simulink library "PropLoads"  (R2024a)
settings: Solver=VariableStepAuto  StartTime=0.0  StopTime=10.0  RelTol=1e-3
undefined symbols (not defined in the file): m1_fail, m2_fail, m3_fail, m4_fail, r1, r2, r3, r4
libraries: matrix_library x4, MT3515 x4, simulink_extras x2, aerolibatmos2 x1, aerolibasang x1
settings Model: Creator=igmso  LastModifiedBy=igmso

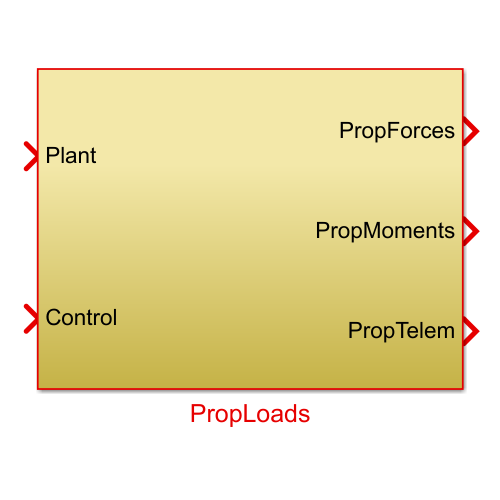
[thumbnail: Simulink's stored preview of the top-level diagram]
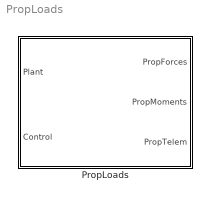
== system PropLoads ==
  PropLoads : Subsystem

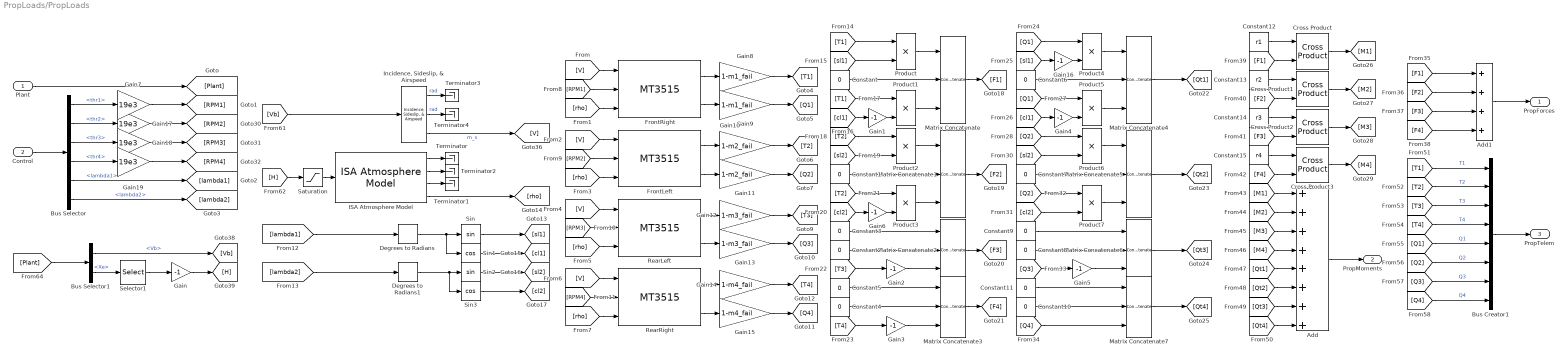
== system PropLoads/PropLoads ==
  Plant : Inport
  Control : Inport  Port=2
  Add : Sum  Inputs=8
  Add1 : Sum  Inputs=4
  Bus Creator1 : BusCreator  Inputs=8
  Bus Selector : BusSelector  OutputSignals=thr1,thr2,thr3,thr4,lambda1,lambda2
  Bus Selector1 : BusSelector  OutputSignals=Vb,Xe
  Constant{,1..11} (12 alike) : Constant  Value=0  SampleTime=-1
  Constant12 : Constant  Value=r1  SampleTime=-1
  Constant13 : Constant  Value=r2  SampleTime=-1
  Constant14 : Constant  Value=r3  SampleTime=-1
  Constant15 : Constant  Value=r4  SampleTime=-1
  Cross Product{,1..3} (4 alike) : matrix_library/Cross Product
  Degrees to Radians : simulink_extras/Transformations/Degrees to Radians
  Degrees to Radians1 : simulink_extras/Transformations/Degrees to Radians
  FrontLeft : MT3515/MT3515  SystemSampleTime=-1  VariantActivationTime=update diagram  AllowFlexibleInterface=on  Latency=0  AutoFrameSizeCalculation=off
  FrontRight : MT3515/MT3515  SystemSampleTime=-1  VariantActivationTime=update diagram  AllowFlexibleInterface=on  Latency=0  AutoFrameSizeCalculation=off
  Gain{,1..6,16} (8 alike) : Gain  Gain=-1
  Gain10 : Gain  Gain=1-m2_fail
  Gain11 : Gain  Gain=1-m2_fail
  Gain12 : Gain  Gain=1-m3_fail
  Gain13 : Gain  Gain=1-m3_fail
  Gain14 : Gain  Gain=1-m4_fail
  Gain15 : Gain  Gain=1-m4_fail
  Gain{7,17..19} (4 alike) : Gain  Gain=19e3
  Gain8 : Gain  Gain=1-m1_fail
  Gain9 : Gain  Gain=1-m1_fail
  ISA Atmosphere Model : aerolibatmos2/ISA Atmosphere Model  useExtended=off  action=Warning  custom=off  viscosityOut=off  g=9.80665  gamma=1.4  R=287.0531  L=0.0065  h_trop=11000  h_strat=20000  rho0=1.225  P0=101325  T0=288.15  h0=0  S=110.4  Tref=273.15  muref=1.716e-5
  "Incidence, Sideslip, & Airspeed" : aerolibasang/Incidence, Sideslip, & Airspeed
  Matrix Concatenate{,1..7} (8 alike) : Concatenate  NumInputs=3  ConcatenateDimension=2
  Product{,1..7} (8 alike) : Product
  RearLeft : MT3515/MT3515  SystemSampleTime=-1  VariantActivationTime=update diagram  AllowFlexibleInterface=on  Latency=0  AutoFrameSizeCalculation=off
  RearRight : MT3515/MT3515  SystemSampleTime=-1  VariantActivationTime=update diagram  AllowFlexibleInterface=on  Latency=0  AutoFrameSizeCalculation=off
  Saturation : Saturate  UpperLimit=20e3  LowerLimit=0
  Selector1 : Selector  InputPortWidth=3  IndexOptions=Index vector (dialog)  Indices=3  OutputSizes=1
  Sin : Trigonometry
  Sin1 : Trigonometry  Operator=cos
  Sin2 : Trigonometry
  Sin3 : Trigonometry  Operator=cos
  Terminator{,1..4} (5 alike) : Terminator
  PropForces : Outport
  PropMoments : Outport  Port=2
  PropTelem : Outport  Port=3
  wires:
  Saturation/1 -> ISA Atmosphere Model/1
  Gain19/1 -> [RPM4]
  Gain18/1 -> [RPM3]
  Gain17/1 -> [RPM2]
  Gain7/1 -> [RPM1]
  Gain16/1 -> Product4/2
  Gain14/1 -> [T4]
  Gain15/1 -> [Q4]
  Gain13/1 -> [Q3]
  Gain12/1 -> [T3]
  Gain11/1 -> [Q2]
  Gain10/1 -> [T2]
  Gain9/1 -> [Q1]
  Gain8/1 -> [T1]
  Product5/1 -> Matrix Concatenate4/3
  [RPM3] -> RearLeft/2
  Cross Product3/1 -> [M4]
  [rho] -> RearLeft/3
  FrontLeft/1 -> Gain10/1
  Constant12/1 -> Cross Product/1
  [T2] -> Product2/1
  [T3] -> Gain2/1
  [lambda2] -> Degrees to Radians1/1
  Sin1/1 -> [cl1]
  Matrix Concatenate1/1 -> [F2]
  [rho] -> FrontLeft/3
  [RPM4] -> RearRight/2
  FrontLeft/2 -> Gain11/1
  [RPM1] -> FrontRight/2
  Matrix Concatenate5/1 -> [Qt2]
  Bus Selector/1 -> Gain7/1  "<thr1>"
  Gain5/1 -> Matrix Concatenate6/3
  Sin3/1 -> [cl2]
  Matrix Concatenate7/1 -> [Qt4]
  [F1] -> Cross Product/2
  [V] -> FrontRight/1
  Gain4/1 -> Product5/2
  [cl2] -> Gain6/1
  [T1] -> Bus Creator1/1  "T1"
  [cl2] -> Product7/2
  [Q1] -> Product4/1
  [Qt3] -> Add/7
  Degrees to Radians1/1 -> Sin3/1, Sin2/1
  [lambda1] -> Degrees to Radians/1
  [sl2] -> Product6/2
  [M4] -> Add/4
  [M2] -> Add/2
  [M1] -> Add/1
  RearRight/1 -> Gain14/1
  [rho] -> RearRight/3
  Product3/1 -> Matrix Concatenate1/3
  [M3] -> Add/3
  [RPM2] -> FrontLeft/2
  [Qt4] -> Add/8
  [T4] -> Gain3/1
  [Qt2] -> Add/6
  [Qt1] -> Add/5
  Matrix Concatenate/1 -> [F1]
  RearLeft/2 -> Gain13/1
  Bus Creator1/1 -> PropTelem/1
  [Q1] -> Product5/1
  Product4/1 -> Matrix Concatenate4/1
  [V] -> RearLeft/1
  [F1] -> Add1/1
  FrontRight/2 -> Gain9/1
  Constant15/1 -> Cross Product3/1
  [V] -> FrontLeft/1
  RearRight/2 -> Gain15/1
  RearLeft/1 -> Gain12/1
  [Q2] -> Product7/1
  Constant4/1 -> Matrix Concatenate3/2
  [V] -> RearRight/1
  Bus Selector/6 -> [lambda2]  "<lambda2>"
  [cl1] -> Gain4/1
  [F2] -> Cross Product1/2
  [T4] -> Bus Creator1/4  "T4"
  [rho] -> FrontRight/3
  Bus Selector/5 -> [lambda1]  "<lambda1>"
  Constant1/1 -> Matrix Concatenate1/2
  Product2/1 -> Matrix Concatenate1/1
  [Q3] -> Gain5/1
  [sl2] -> Product2/2
  Plant/1 -> [Plant]
  Cross Product2/1 -> [M3]
  [cl1] -> Gain1/1
  [T2] -> Product3/1
  Constant11/1 -> Matrix Concatenate7/1
  Degrees to Radians/1 -> Sin1/1, Sin/1
  Constant10/1 -> Matrix Concatenate7/2
  [Q4] -> Bus Creator1/8  "Q4"
  Matrix Concatenate6/1 -> [Qt3]
  Matrix Concatenate3/1 -> [F4]
  [Q4] -> Matrix Concatenate7/3
  Constant9/1 -> Matrix Concatenate6/1
  Constant8/1 -> Matrix Concatenate6/2
  Product6/1 -> Matrix Concatenate5/1
  [Q2] -> Product6/1
  Constant7/1 -> Matrix Concatenate5/2
  Matrix Concatenate4/1 -> [Qt1]
  Product7/1 -> Matrix Concatenate5/3
  [sl1] -> Gain16/1
  Constant6/1 -> Matrix Concatenate4/2
  [T1] -> Product1/1
  Add/1 -> PropMoments/1
  Product/1 -> Matrix Concatenate/1
  [F3] -> Cross Product2/2
  Constant/1 -> Matrix Concatenate/2
  Product1/1 -> Matrix Concatenate/3
  Gain3/1 -> Matrix Concatenate3/3
  Constant14/1 -> Cross Product2/1
  Constant5/1 -> Matrix Concatenate3/1
  [T2] -> Bus Creator1/2  "T2"
  [T3] -> Bus Creator1/3  "T3"
  [Q2] -> Bus Creator1/6  "Q2"
  [Q1] -> Bus Creator1/5  "Q1"
  [Q3] -> Bus Creator1/7  "Q3"
  Cross Product/1 -> [M1]
  [T1] -> Product/1
  [F4] -> Cross Product3/2
  FrontRight/1 -> Gain8/1
  [sl1] -> Product/2
  Gain1/1 -> Product1/2
  [F2] -> Add1/2
  [F3] -> Add1/3
  [F4] -> Add1/4
  Cross Product1/1 -> [M2]
  Sin/1 -> [sl1]
  Constant3/1 -> Matrix Concatenate2/1
  Constant2/1 -> Matrix Concatenate2/2
  Matrix Concatenate2/1 -> [F3]
  Sin2/1 -> [sl2]
  Constant13/1 -> Cross Product1/1
  Add1/1 -> PropForces/1
  Gain2/1 -> Matrix Concatenate2/3
  Control/1 -> Bus Selector/1
  Bus Selector/2 -> Gain17/1  "<thr2>"
  Bus Selector/3 -> Gain18/1  "<thr3>"
  Bus Selector/4 -> Gain19/1  "<thr4>"
  Gain6/1 -> Product3/2
  "Incidence, Sideslip, & Airspeed"/1 -> Terminator3/1  "rad"
  "Incidence, Sideslip, & Airspeed"/2 -> Terminator4/1  "rad"
  [H] -> Saturation/1
  ISA Atmosphere Model/2 -> Terminator2/1
  "Incidence, Sideslip, & Airspeed"/3 -> [V]  "m_s"
  ISA Atmosphere Model/3 -> Terminator1/1
  ISA Atmosphere Model/1 -> Terminator/1
  [Vb] -> "Incidence, Sideslip, & Airspeed"/1
  Gain/1 -> [H]
  [Plant] -> Bus Selector1/1
  Bus Selector1/1 -> [Vb]  "<Vb>"
  Selector1/1 -> Gain/1
  Bus Selector1/2 -> Selector1/1  "<Xe>"
  ISA Atmosphere Model/4 -> [rho]
